simulink subsystem "Wind_Model"  (R2023b)
settings: Solver=VariableStepAuto  StartTime=0.0  StopTime=10.0  RelTol=1e-3
undefined symbols (not defined in the file): F, Light, MIL, time0, wind_direction, wind_speed
libraries: sharedtransform x1, aerolibwind2 x1
settings Model: Creator=thatf  LastModifiedBy=thatf

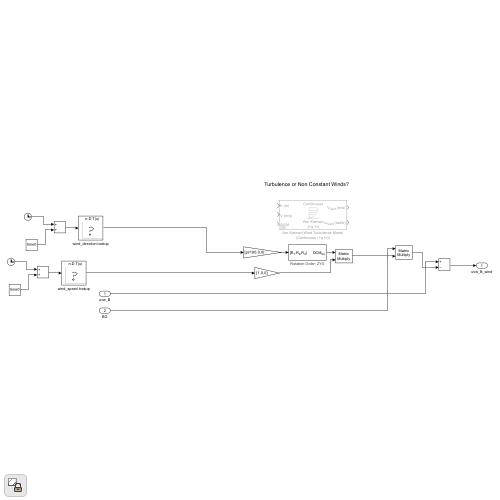
[thumbnail: Simulink's stored preview of the top-level diagram]
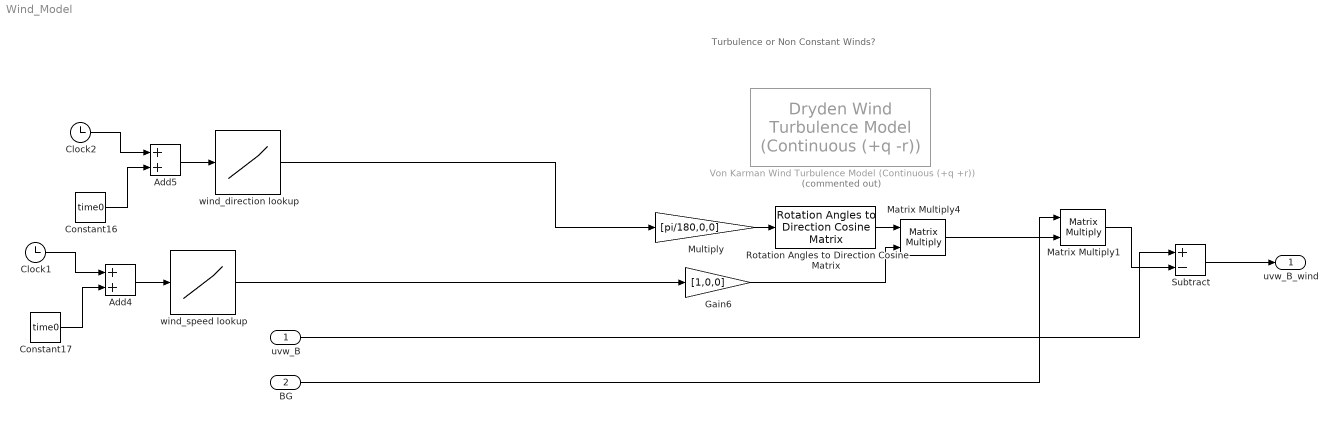
== system Wind_Model ==
  note: Turbulence or Non Constant Winds?
  uvw_B : Inport
  BG : Inport  Port=2
  Add4 : Sum
  Add5 : Sum
  Clock1 : Clock
  Clock2 : Clock
  Constant16 : Constant  Value=time0
  Constant17 : Constant  Value=time0
  Gain6 : Gain  Gain=[1,0,0]
  Matrix Multiply1 : Product  Multiplication=Matrix(*)
  Matrix Multiply4 : Product  Multiplication=Matrix(*)
  Multiply : Gain  Gain=[pi/180,0,0]
  Rotation Angles to Direction Cosine Matrix : sharedtransform/Rotation Angles to Direction Cosine Matrix  rotationOrder=ZYX  aMode=aMode
  Subtract : Sum  Inputs=+-
  Von Karman Wind Turbulence Model (Continuous (+q +r)) : aerolibwind2/Dryden Wind Turbulence Model  (Continuous (+q -r))  Commented=on  units=Metric (MKS)  spec=MIL-F-8785C  model=Continuous Von Karman (+q +r)  W20=15  Wdeg=0  TurbProb=10^-2 - Light  L_high=762  Wingspan=10  ts=0.1  Seed=[23341 23342 23343 23344]  T_on=on
      settings: LibrarySourceBlock=|
      | aerolibwind2/Von Karman Wind Turbulence Model
      | (Continuous (+q +r))
  wind_direction lookup : Lookup_n-D  NumberOfTableDimensions=1  BreakpointsForDimension1=wind_direction(:,1)  Table=wind_direction(:,2)  InternalRulePriority=Speed  RndMeth=Simplest
  wind_speed lookup : Lookup_n-D  NumberOfTableDimensions=1  BreakpointsForDimension1=wind_speed(:,1)  Table=wind_speed(:,2)  InternalRulePriority=Speed  RndMeth=Simplest
  uvw_B_wind : Outport
  wires:
  Rotation Angles to Direction Cosine Matrix/1 -> Matrix Multiply4/1
  BG/1 -> Matrix Multiply1/1
  Gain6/1 -> Matrix Multiply4/2
  Multiply/1 -> Rotation Angles to Direction Cosine Matrix/1
  uvw_B/1 -> Subtract/1
  Matrix Multiply4/1 -> Matrix Multiply1/2
  Matrix Multiply1/1 -> Subtract/2
  Subtract/1 -> uvw_B_wind/1
  Constant17/1 -> Add4/2
  wind_speed lookup/1 -> Gain6/1
  wind_direction lookup/1 -> Multiply/1
  Add5/1 -> wind_direction lookup/1
  Add4/1 -> wind_speed lookup/1
  Constant16/1 -> Add5/2
  Clock2/1 -> Add5/1
  Clock1/1 -> Add4/1
